simulink model "generic_truck"  (R2025a)
settings: Solver=VariableStepAuto  StartTime=0.0  StopTime=600  FixedStep=0.01  MaxStep=0.001  RelTol=1e-3  EnableMultiTasking=on
libraries: TruckMaker4SL x205, simulink x1
(part 8 of 9)

== matlab function generic_truck/TruckMaker/Tractor_Subsystem /ONE_TRACK_MODEL_TRACTOR_UKF/MATLAB Function1 ==
  data: z input; u input; xhat output; Q input; R input; Ts input; data input; P output; dxdt output; innovation output; K_out output; S_out output; z_pred_out output
function [xhat, P, dxdt, innovation, K_out, S_out, z_pred_out] = UKF_OneTrack_IMU(z, u, Q, R, Ts,data)

persistent x Pk dxdt_old t p_nom Pp

if isempty(x)
    x = [15;0.1;0.1;7.5;7.5];
end
if isempty(Pk)
    Pk = diag([0.1 0.1 0.1 5 5]);
end
if isempty(dxdt_old)
    dxdt_old = zeros(5,1);
end
if isempty(t)
    t = 0;
end
if isempty(p_nom)
    p_nom = [6800; 12994.917];
    Pp = diag([5000, 20000]).^2;
end

T_sim = 0.001;
t = t + T_sim;
t=data;

if t < 30
    xhat = x;
    P = Pk;
    dxdt = dxdt_old;
    innovation = zeros(length(z),1);
    K_out = zeros(length(x), length(z));
    S_out = eye(length(z));
    z_pred_out = zeros(length(z),1);
    return
end

IDX_VX  = 3; 
IDX_WRL = 6; 
IDX_WRR = 7;

g  = 9.82;

p_cog = [3.473;0;0.925];
p_fax = [4.520;0;0.490];
p_rax = [0.950;0;0.490];
p_imu = [3.600;0;1.000];

lf = abs(p_fax(1)-p_cog(1));
lr = abs(p_cog(1)-p_rax(1));
L  = lf + lr;
h  = p_cog(3);

Rfax = p_fax - p_cog; Rfax(3) = -p_cog(3);
Rrax = p_rax - p_cog; Rrax(3) = -p_cog(3);
Rcog = p_imu - p_cog;

delta = u(1);
T_rl  = u(2);
T_rr  = u(3);
Rwheel = 0.505;
Fx_vehicle = (T_rl + T_rr)/Rwheel;

n  = length(x);
np = length(p_nom);
nSPx = 2*n + 1;
nSPp = 2*np;
nSP  = nSPx + nSPp;

W0 = 1 - (n + np)/3;
Wi = (1 - W0)/(2*(n + np));
gamma = sqrt((n + np)/(1 - W0));

%% ===== STATE SIGMA =====
Pk = (Pk + Pk')/2 + 1e-9*eye(n);
Sx = chol(Pk,'lower');

X = zeros(n,nSPx);
X(:,1) = x;
for i=1:n
    X(:,i+1)   = x + gamma*Sx(:,i);
    X(:,i+1+n) = x - gamma*Sx(:,i);
end

%% ===== PARAM SIGMA =====
Pp = (Pp + Pp')/2 + 1e-9*eye(np);
Sp = chol(Pp,'lower');

SPp = zeros(np,nSPp);
for i=1:np
    SPp(:,i)    = p_nom + gamma*Sp(:,i);
    SPp(:,i+np) = p_nom - gamma*Sp(:,i);
end

%% ===== PREDICTION =====
X_prop = zeros(n,nSP);
dxdt_model = zeros(5,1);

for k=1:nSP
    if k <= nSPx
        Xk = X(:,k); 
        pk = p_nom;
    else
        Xk = x; 
        pk = SPp(:,k-nSPx);
    end

    vx=Xk(1); vy=Xk(2); wz=Xk(3); Cf=Xk(4); Cr=Xk(5);
    m=pk(1); Jz=pk(2);

    v_cog=[vx;vy;0]; 
    omega=[0;0;wz];

    Rotf=[cos(delta) -sin(delta) 0;
          sin(delta)  cos(delta)  0; 
           0          0          1];

    vf=Rotf.'*(v_cog+cross(omega,Rfax));
    vr=v_cog+cross(omega,Rrax);

    alpha_f=atan2(vf(2),max(abs(vf(1)),0.1));
    alpha_r=atan2(vr(2),max(abs(vr(1)),0.1));

    ax_est=Fx_vehicle/m+vy*wz;

    Ffz=m*g*lr/L - m*ax_est*h/L;
    Frz=m*g*lf/L + m*ax_est*h/L;

    Fy_f=-Cf*alpha_f*Ffz;
    Fy_r=-Cr*alpha_r*Frz;

    dvx=(Fx_vehicle - Fy_f*sin(delta))/m + vy*wz;
    dvy=(Fy_f*cos(delta)+Fy_r)/m - vx*wz;
    dwz=(lf*Fy_f*cos(delta) - lr*Fy_r)/Jz;

    if k==1
        dxdt_model=[dvx;dvy;dwz;0;0];
    end

    X_prop(:,k)=[vx+Ts*dvx; vy+Ts*dvy; wz+Ts*dwz; Cf; Cr];
end

%% ===== MEAN =====
x_pred=zeros(n,1);
for k=1:nSP
    w=(k==1)*W0 + (k>1)*Wi;
    x_pred=x_pred + w*X_prop(:,k);
end

%% ===== COV =====
P_pred=zeros(n);
for k=1:nSPx
    w=(k==1)*W0 + (k>1)*Wi;
    dx=X_prop(:,k)-x_pred;
    P_pred=P_pred + w*(dx*dx');
end
P_pred=P_pred + Q*Ts;

%% ===== NEW SIGMA POINTS =====
P_pred=(P_pred+P_pred')/2 + 1e-9*eye(n);
Sx=chol(P_pred,'lower');

SPx_new=zeros(n,nSPx);
SPx_new(:,1)=x_pred;

for i=1:n
    SPx_new(:,i+1)  =x_pred+gamma*Sx(:,i);
    SPx_new(:,i+1+n) =x_pred-gamma*Sx(:,i);
end

%% ===== MEASUREMENT =====
Z=zeros(length(z),nSP);

for k=1:nSP
    if k<=nSPx
        Xk=SPx_new(:,k);
        pk=p_nom;
    else
        Xk=x_pred;
        pk=SPp(:,k-nSPx);
    end

    vx=Xk(1); vy=Xk(2); wz=Xk(3);
    Cf=Xk(4); Cr=Xk(5);

    m=pk(1); Jz=pk(2);

    v_cog=[vx;vy;0]; omega=[0;0;wz];
    Rotf=[cos(delta) -sin(delta) 0; sin(delta) cos(delta) 0; 0 0 1];

    vf=Rotf.'*(v_cog+cross(omega,Rfax));
    vr=v_cog+cross(omega,Rrax);

    alpha_f=atan2(vf(2),max(abs(vf(1)),0.1));
    alpha_r=atan2(vr(2),max(abs(vr(1)),0.1));

    ax_est=Fx_vehicle/m+vy*wz;

    Ffz=m*g*lr/L - m*ax_est*h/L;
    Frz=m*g*lf/L + m*ax_est*h/L;

    Fy_f=-Cf*alpha_f*Ffz;
    Fy_r=-Cr*alpha_r*Frz;

    dvx=(Fx_vehicle - Fy_f*sin(delta))/m;
    dvy=(Fy_f*cos(delta)+Fy_r)/m;
    dwz=(lf*Fy_f*cos(delta) - lr*Fy_r)/Jz;

    a_cog=[dvx;dvy;0];
    alpha_vec=[0;0;dwz];

    a_imu=a_cog + cross(omega,cross(omega,Rcog)) + cross(alpha_vec,Rcog);
    v_imu=v_cog + cross(omega,Rcog);

    omega_rl=vx/Rwheel;
    omega_rr=vx/Rwheel;

    Z(:,k)=[a_imu(1:2); v_imu(1:2); wz; omega_rl; omega_rr];
end

%% ===== z mean =====
z_pred=zeros(length(z),1);
for k=1:nSP
    w=(k==1)*W0 + (k>1)*Wi;
    z_pred=z_pred + w*Z(:,k);
end

%% ===== SENSOR SELECTION =====
valid_idx=true(length(z),1);

if ~isnan(z(IDX_VX))
    valid_idx(IDX_WRL)=false;
    valid_idx(IDX_WRR)=false;
else
    valid_idx(IDX_VX)=false;
end

valid_idx=valid_idx & ~isnan(z);

z_used=z(valid_idx);
z_pred_used=z_pred(valid_idx);
Z_used=Z(valid_idx,:);
R_used=R(valid_idx,valid_idx);

%% ===== S =====
S_cov=zeros(length(z_used));
for k=1:nSP
    w=(k==1)*W0 + (k>1)*Wi;
    dz=Z_used(:,k)-z_pred_used;
    S_cov=S_cov + w*(dz*dz');
end

S_cov=S_cov + R_used;
S_cov=(S_cov+S_cov')/2 + 1e-9*eye(size(S_cov));

%% ===== Pxz =====
Pxz=zeros(n,length(z_used));
for k=1:nSPx
    w=(k==1)*W0 + (k>1)*Wi;
    dx=SPx_new(:,k)-x_pred;
    dz=Z_used(:,k)-z_pred_used;
    Pxz=Pxz + w*(dx*dz');
end

%% ===== UPDATE =====
K=Pxz/S_cov;

x=x_pred + K*(z_used - z_pred_used);
Pk=P_pred - K*S_cov*K';
Pk=(Pk+Pk')/2 + 1e-9*eye(n);

%% ===== OUTPUT =====
xhat=x;
P=Pk;
dxdt=dxdt_model;

innovation=zeros(length(z),1);
innovation(valid_idx)=z_used - z_pred_used;

K_out=zeros(n,length(z));
K_out(:,valid_idx)=K;

S_out=zeros(length(z));
S_out(valid_idx,valid_idx)=S_cov;

z_pred_out=z_pred;

end

== matlab function generic_truck/TruckMaker/Tractor_Subsystem /ONE_TRACK_MODEL_TRACTOR_UKF/MATLAB Function2 ==
  data: z input; u input; Q input; R input; Ts input; xhat output; data input; P output; dxdt output; innovation output; K_out output; S_out output; z_pred_out output
function [xhat, P, dxdt, innovation, K_out, S_out, z_pred_out] = UKF_OneTrack_IMU(z, u, Q, R, Ts, data)
z=z(1:5);
persistent x Pk dxdt_old t

%% =========================
%% INIT
%% =========================
if isempty(x)
    % [vx vy wz Cf Cr bax]
    x = [15;0.1;0.1;7.5;7.5;0];
end

if isempty(Pk)
    Pk = diag([0.1 0.1 0.1 5 5 0.5]);
end

if isempty(dxdt_old)
    dxdt_old = zeros(6,1);
end

if isempty(t)
    t = 0;
end

t = data;

if t < 30
    xhat = x;
    P = Pk;
    dxdt = dxdt_old;
    innovation = zeros(length(z),1);
    K_out = zeros(length(x), length(z));
    S_out = eye(length(z));
    z_pred_out = zeros(length(z),1);
    return
end

IDX_VX = 3;
IDX_VY = 4;

%% =========================
%% VEHICLE CONSTANTS
%% =========================
g  = 9.82;

p_cog = [3.473;0;0.925];
p_fax = [4.520;0;0.490];
p_rax = [0.950;0;0.490];
p_imu = [3.600;0;1.000];

lf = abs(p_fax(1)-p_cog(1));
lr = abs(p_cog(1)-p_rax(1));
L  = lf + lr;
h  = p_cog(3);

Rfax = p_fax - p_cog; Rfax(3) = -p_cog(3);
Rrax = p_rax - p_cog; Rrax(3) = -p_cog(3);
Rcog = p_imu - p_cog;

%% =========================
%% INPUTS
%% =========================
delta = u(1);
T_rl  = u(2);
T_rr  = u(3);
Rwheel = 0.505;
Fx_vehicle = (T_rl + T_rr)/Rwheel;

%% =========================
%% UKF PARAMS
%% =========================
n = length(x);
nSPx = 2*n + 1;

W0 = 1 - n/3;
Wi = (1 - W0)/(2*n);
gamma = sqrt(n/(1-W0));

%% =========================
%% SIGMA POINTS (PRIOR)
%% =========================
Pk = (Pk + Pk')/2 + 1e-9*eye(n);
Sx = chol(Pk,'lower');

X_pre = zeros(n,nSPx);
X_pre(:,1) = x;

for i=1:n
    X_pre(:,i+1)   = x + gamma*Sx(:,i);
    X_pre(:,i+1+n) = x - gamma*Sx(:,i);
end

%% =========================
%% PREDICTION
%% =========================
X_pred = zeros(n,nSPx);
dxdt_model = zeros(n,1);

m = 6800; 
Jz = 12994.917;

for k=1:nSPx

    Xk = X_pre(:,k);

    vx = Xk(1); vy = Xk(2); wz = Xk(3);
    Cf = Xk(4); Cr = Xk(5);
    bax = Xk(6);

    v_cog = [vx; vy; 0]; 
    omega = [0; 0; wz];

    Rotf = [cos(delta) -sin(delta) 0;
            sin(delta)  cos(delta) 0;
            0 0 1];

    vf = Rotf.'*(v_cog + cross(omega,Rfax));
    vr = v_cog + cross(omega,Rrax);

    alpha_f = atan2(vf(2), max(abs(vf(1)),0.1));
    alpha_r = atan2(vr(2), max(abs(vr(1)),0.1));

    ax_est = Fx_vehicle/m + vy*wz;

    Ffz = m*g*lr/L - m*ax_est*h/L;
    Frz = m*g*lf/L + m*ax_est*h/L;

    Fy_f = -Cf*alpha_f*Ffz;
    Fy_r = -Cr*alpha_r*Frz;

    dvx = (Fx_vehicle - Fy_f*sin(delta))/m + vy*wz + bax;

    % Testa DÄMPNING här (NYCKELN!)
    dvy = (Fy_f*cos(delta)+Fy_r)/m - vx*wz;

    dwz = (lf*Fy_f*cos(delta) - lr*Fy_r)/Jz;

    if k==1
        dxdt_model = [dvx; dvy; dwz; 0; 0; 0];
    end

    X_pred(:,k) = [
        vx + Ts*dvx
        vy + Ts*dvy
        wz + Ts*dwz
        Cf
        Cr
        bax
    ];
end

%% =========================
%% MEAN
%% =========================
x_pred = zeros(n,1);
for k=1:nSPx
    w = (k==1)*W0 + (k>1)*Wi;
    x_pred = x_pred + w*X_pred(:,k);
end

%% =========================
%% COVARIANCE
%% =========================
P_pred = zeros(n);
for k=1:nSPx
    w = (k==1)*W0 + (k>1)*Wi;
    dx = X_pred(:,k) - x_pred;
    P_pred = P_pred + w*(dx*dx');
end

P_pred = P_pred + Q*Ts;
P_pred = (P_pred + P_pred')/2 + 1e-9*eye(n);

%% =========================
%% SIGMA POINTS (POST)
%% =========================
Sx = chol(P_pred,'lower');

X_post = zeros(n,nSPx);
X_post(:,1) = x_pred;

for i=1:n
    X_post(:,i+1)   = x_pred + gamma*Sx(:,i);
    X_post(:,i+1+n) = x_pred - gamma*Sx(:,i);
end

%% =========================
%% MEASUREMENT MODEL
%% =========================
Z = zeros(length(z), nSPx);

for k=1:nSPx

    Xk = X_post(:,k);

    vx = Xk(1); vy = Xk(2); wz = Xk(3);
    Cf = Xk(4); Cr = Xk(5);
    bax = Xk(6);

    v_cog = [vx; vy; 0]; 
    omega=[0;0;wz];

    Rotf=[cos(delta) -sin(delta) 0;
          sin(delta)  cos(delta) 0;
          0 0 1];

    vf = Rotf.'*(v_cog+cross(omega,Rfax));
    vr = v_cog+cross(omega,Rrax);

    alpha_f = atan2(vf(2), max(abs(vf(1)),0.1));
    alpha_r = atan2(vr(2), max(abs(vr(1)),0.1));

    ax_est = Fx_vehicle/m + vy*wz;

    Ffz = m*g*lr/L - m*ax_est*h/L;
    Frz = m*g*lf/L + m*ax_est*h/L;

    Fy_f = -Cf*alpha_f*Ffz;
    Fy_r = -Cr*alpha_r*Frz;
    
    dvx = (Fx_vehicle - Fy_f*sin(delta))/m;
    dvy = (Fy_f*cos(delta)+Fy_r)/m;
    dwz = (lf*Fy_f*cos(delta) - lr*Fy_r)/Jz;

    a_cog = [dvx; dvy; 0];
    alpha_vec=[0;0;dwz];

    a_imu = a_cog + cross(omega,cross(omega,Rcog)) + cross(alpha_vec,Rcog);
    v_imu = v_cog + cross(omega,Rcog);

    ax_meas = a_imu(1) + bax;

    Z(:,k) = [
        ax_meas
        a_imu(2)
        v_imu(1:2)
        wz
    ];
end

%% =========================
%% MEASUREMENT MEAN
%% =========================
z_pred = zeros(length(z),1);
for k=1:nSPx
    w = (k==1)*W0 + (k>1)*Wi;
    z_pred = z_pred + w*Z(:,k);
end

%% =========================
%% SENSOR SELECTION
%% =========================
valid_idx = true(length(z),1);

if isnan(z(IDX_VX))
    valid_idx(IDX_VX) = false;
    valid_idx(IDX_VY) = false;
end

valid_idx = valid_idx & ~isnan(z);

z_used = z(valid_idx);
z_pred_used = z_pred(valid_idx);
Z_used = Z(valid_idx,:);
R_used = R(valid_idx,valid_idx);

%% =========================
%% S + Pxz
%% =========================
S_cov = zeros(length(z_used));
Pxz = zeros(n,length(z_used));

for k=1:nSPx
    w = (k==1)*W0 + (k>1)*Wi;

    dz = Z_used(:,k)-z_pred_used;
    dx = X_post(:,k)-x_pred;

    S_cov = S_cov + w*(dz*dz');
    Pxz = Pxz + w*(dx*dz');
end

S_cov = S_cov + R_used;
S_cov = (S_cov + S_cov')/2 + 1e-9*eye(size(S_cov));

%% =========================
%% UPDATE
%% =========================
K = Pxz / S_cov;

x = x_pred + K*(z_used - z_pred_used);
Pk = P_pred - K*S_cov*K';
Pk = (Pk + Pk')/2 + 1e-9*eye(n);

%% =========================
%% OUTPUT
%% =========================
xhat = x;
P = Pk;
dxdt = dxdt_model;

innovation = zeros(length(z),1);
innovation(valid_idx) = z_used - z_pred_used;

K_out = zeros(n,length(z));
K_out(:,valid_idx) = K;

S_out = zeros(length(z));
S_out(valid_idx,valid_idx) = S_cov;

z_pred_out = z_pred;

end

== matlab function generic_truck/TruckMaker/Tractor_Subsystem /ONE_TRACK_MODEL_TRACTOR_UKF/UKF_ONE_TRACK1 ==
  data: z input; u input; xhat output; Q input; R input; Ts input; P output; dxdt output; innovation output; K_out output; S_out output; z_pred_out output; data input
function [xhat, P, dxdt, innovation, K_out, S_out, z_pred_out] = UKF_OneTrack_IMU(z, u, Q, R, Ts,data)

persistent x Pk dxdt_old t p_nom Pp

if isempty(x)
    x = [15;0.1;0.1;7.5;7.5];
end
if isempty(Pk)
    Pk = diag([0.1 0.1 0.1 5 5]);
end
if isempty(dxdt_old)
    dxdt_old = zeros(5,1);
end
if isempty(t)
    t = 0;
end
if isempty(p_nom)
    p_nom = [6800; 12994.917];
    Pp = diag([5000, 20000]).^2;
end

T_sim = 0.001;
t = t + T_sim;
t=data;

if t < 49.9
    xhat = x;
    P = Pk;
    dxdt = dxdt_old;
    innovation = zeros(length(z),1);
    K_out = zeros(length(x), length(z));
    S_out = eye(length(z));
    z_pred_out = zeros(length(z),1);
    return
end

IDX_VX  = 3; 
IDX_WRL = 6; 
IDX_WRR = 7;

g  = 9.82;

p_cog = [3.473;0;0.925];
p_fax = [4.520;0;0.490];
p_rax = [0.950;0;0.490];
p_imu = [3.600;0;1.000];

lf = abs(p_fax(1)-p_cog(1));
lr = abs(p_cog(1)-p_rax(1));
L  = lf + lr;
h  = p_cog(3);

Rfax = p_fax - p_cog; Rfax(3) = -p_cog(3);
Rrax = p_rax - p_cog; Rrax(3) = -p_cog(3);
Rcog = p_imu - p_cog;

delta = u(1);
T_rl  = u(2);
T_rr  = u(3);
F_brake= abs(u(4)) + abs(u(5));
Rwheel = 0.505;
Fx_vehicle = (T_rl + T_rr)/Rwheel - F_brake;

n  = length(x);
np = length(p_nom);
nSPx = 2*n + 1;
nSPp = 2*np;
nSP  = nSPx + nSPp;

W0 = 1 - (n + np)/3;
Wi = (1 - W0)/(2*(n + np));
gamma = sqrt((n + np)/(1 - W0));

%% ===== STATE SIGMA =====
Pk = (Pk + Pk')/2 + 1e-9*eye(n);
Sx = chol(Pk,'lower');

X = zeros(n,nSPx);
X(:,1) = x;
for i=1:n
    X(:,i+1)   = x + gamma*Sx(:,i);
    X(:,i+1+n) = x - gamma*Sx(:,i);
end

%% ===== PARAM SIGMA =====
Pp = (Pp + Pp')/2 + 1e-9*eye(np);
Sp = chol(Pp,'lower');

SPp = zeros(np,nSPp);
for i=1:np
    SPp(:,i)    = p_nom + gamma*Sp(:,i);
    SPp(:,i+np) = p_nom - gamma*Sp(:,i);
end

%% ===== PREDICTION =====
X_prop = zeros(n,nSP);
dxdt_model = zeros(5,1);

for k=1:nSP
    if k <= nSPx
        Xk = X(:,k); 
        pk = p_nom;
    else
        Xk = x; 
        pk = SPp(:,k-nSPx);
    end

    vx=Xk(1); vy=Xk(2); wz=Xk(3); Cf=Xk(4); Cr=Xk(5);
    m=pk(1); Jz=pk(2);

    v_cog=[vx;vy;0]; omega=[0;0;wz];
    Rotf=[cos(delta) -sin(delta) 0; sin(delta) cos(delta) 0; 0 0 1];

    vf=Rotf.'*(v_cog+cross(omega,Rfax));
    vr=v_cog+cross(omega,Rrax);

    alpha_f=atan2(vf(2),max(abs(vf(1)),0.1));
    alpha_r=atan2(vr(2),max(abs(vr(1)),0.1));

    ax_est=Fx_vehicle/m+vy*wz;

    Ffz=m*g*lr/L - m*ax_est*h/L;
    Frz=m*g*lf/L + m*ax_est*h/L;

    Fy_f=-Cf*alpha_f*Ffz;
    Fy_r=-Cr*alpha_r*Frz;

    dvx=(Fx_vehicle - Fy_f*sin(delta))/m + vy*wz;
    dvy=(Fy_f*cos(delta)+Fy_r)/m - vx*wz;
    dwz=(lf*Fy_f*cos(delta) - lr*Fy_r)/Jz;

    if k==1
        dxdt_model=[dvx;dvy;dwz;0;0];
    end

    X_prop(:,k)=[vx+Ts*dvx; vy+Ts*dvy; wz+Ts*dwz; Cf; Cr];
end

%% ===== MEAN =====
x_pred=zeros(n,1);
for k=1:nSP
    w=(k==1)*W0 + (k>1)*Wi;
    x_pred=x_pred + w*X_prop(:,k);
end

%% ===== COV =====
P_pred=zeros(n);
for k=1:nSPx
    w=(k==1)*W0 + (k>1)*Wi;
    dx=X_prop(:,k)-x_pred;
    P_pred=P_pred + w*(dx*dx');
end
P_pred=P_pred + Q*Ts;

%% ===== NEW SIGMA POINTS =====
P_pred=(P_pred+P_pred')/2 + 1e-9*eye(n);
Sx=chol(P_pred,'lower');

SPx_new=zeros(n,nSPx);
SPx_new(:,1)=x_pred;

for i=1:n
    SPx_new(:,i+1)=x_pred+gamma*Sx(:,i);
    SPx_new(:,i+1+n)=x_pred-gamma*Sx(:,i);
end

%% ===== MEASUREMENT =====
Z=zeros(length(z),nSP);

for k=1:nSP
    if k<=nSPx
        Xk=SPx_new(:,k);
        pk=p_nom;
    else
        Xk=x_pred;
        pk=SPp(:,k-nSPx);
    end

    vx=Xk(1); vy=Xk(2); wz=Xk(3);
    Cf=Xk(4); Cr=Xk(5);

    m=pk(1); Jz=pk(2);

    v_cog=[vx;vy;0]; omega=[0;0;wz];
    Rotf=[cos(delta) -sin(delta) 0; sin(delta) cos(delta) 0; 0 0 1];

    vf=Rotf.'*(v_cog+cross(omega,Rfax));
    vr=v_cog+cross(omega,Rrax);

    alpha_f=atan2(vf(2),max(abs(vf(1)),0.1));
    alpha_r=atan2(vr(2),max(abs(vr(1)),0.1));

    ax_est=Fx_vehicle/m+vy*wz;

    Ffz=m*g*lr/L - m*ax_est*h/L;
    Frz=m*g*lf/L + m*ax_est*h/L;

    Fy_f=-Cf*alpha_f*Ffz;
    Fy_r=-Cr*alpha_r*Frz;

    dvx=(Fx_vehicle - Fy_f*sin(delta))/m;
    dvy=(Fy_f*cos(delta)+Fy_r)/m;
    dwz=(lf*Fy_f*cos(delta) - lr*Fy_r)/Jz;

    a_cog=[dvx;dvy;0];
    alpha_vec=[0;0;dwz];

    a_imu=a_cog + cross(omega,cross(omega,Rcog)) + cross(alpha_vec,Rcog);
    v_imu=v_cog + cross(omega,Rcog);

    omega_rl=vx/Rwheel;
    omega_rr=vx/Rwheel;

    Z(:,k)=[a_imu(1:2); v_imu(1:2); wz; omega_rl; omega_rr];
end

%% ===== z mean =====
z_pred=zeros(length(z),1);
for k=1:nSP
    w=(k==1)*W0 + (k>1)*Wi;
    z_pred=z_pred + w*Z(:,k);
end

%% ===== SENSOR SELECTION =====
valid_idx=true(length(z),1);

if ~isnan(z(IDX_VX))
    valid_idx(IDX_WRL)=false;
    valid_idx(IDX_WRR)=false;
else
    valid_idx(IDX_VX)=false;
end

valid_idx=valid_idx & ~isnan(z);

z_used=z(valid_idx);
z_pred_used=z_pred(valid_idx);
Z_used=Z(valid_idx,:);
R_used=R(valid_idx,valid_idx);

%% ===== S =====
S_cov=zeros(length(z_used));
for k=1:nSP
    w=(k==1)*W0 + (k>1)*Wi;
    dz=Z_used(:,k)-z_pred_used;
    S_cov=S_cov + w*(dz*dz');
end

S_cov=S_cov + R_used;
S_cov=(S_cov+S_cov')/2 + 1e-9*eye(size(S_cov));

%% ===== Pxz =====
Pxz=zeros(n,length(z_used));
for k=1:nSPx
    w=(k==1)*W0 + (k>1)*Wi;
    dx=SPx_new(:,k)-x_pred;
    dz=Z_used(:,k)-z_pred_used;
    Pxz=Pxz + w*(dx*dz');
end

%% ===== UPDATE =====
K=Pxz/S_cov;

x=x_pred + K*(z_used - z_pred_used);
Pk=P_pred - K*S_cov*K';
Pk=(Pk+Pk')/2 + 1e-9*eye(n);

%% ===== OUTPUT =====
xhat=x;
P=Pk;
dxdt=dxdt_model;

innovation=zeros(length(z),1);
innovation(valid_idx)=z_used - z_pred_used;

K_out=zeros(n,length(z));
K_out(:,valid_idx)=K;

S_out=zeros(length(z));
S_out(valid_idx,valid_idx)=S_cov;

z_pred_out=z_pred;

end

== matlab function generic_truck/TruckMaker/Tractor_Subsystem /ONE_TRACK_MODEL_TRACTOR_UKF/Working Model with 5 measurements  ==
  data: z input; u input; xhat output; Q input; R input; Ts input; P output; dxdt output; innovation output; K_out output; S_out output; z_pred_out output
function [xhat, P, dxdt, innovation, K_out, S_out, z_pred_out] = UKF_OneTrack_IMU(z, u, Q, R, Ts)

% z = [ax; ay; vx; vy; wz]

%% =========================
%% PERSISTENT VARIABLES
%% =========================
persistent x Pk dxdt_old t

if isempty(x)
    x = [15;0.1;0.1;7.5;7.5];   % [vx vy wz Cf Cr]
end
if isempty(Pk)
    Pk = diag([0.1 0.1 0.1 2 2]);
end
if isempty(dxdt_old)
    dxdt_old = zeros(5,1);
end
if isempty(t)
    t = 0;
end

%% =========================
%% TIME UPDATE
%% =========================
t = t + 0.001;

start_time = 30;
if t < start_time
    xhat = x;
    P = Pk;
    dxdt = dxdt_old;

    innovation = zeros(length(z),1);
    K_out = zeros(length(x), length(z));
    S_out = eye(length(z));
    z_pred_out = zeros(length(z),1);
    return
end

%% =========================
%% VEHICLE PARAMETERS
%% =========================
m  = 6800;
g  = 9.82;
Jz = 12994.917;

p_cog = [3.473;0;0.925];
p_fax = [4.520;0;0.490];
p_rax = [0.950;0;0.490];
p_imu = [3.600;0;1.000];

lf = abs(p_fax(1)-p_cog(1));
lr = abs(p_cog(1)-p_rax(1));
L  = lf + lr;
h  = p_cog(3);

Rfax = p_fax - p_cog; Rfax(3) = -p_cog(3);
Rrax = p_rax - p_cog; Rrax(3) = -p_cog(3);
Rcog = p_imu - p_cog;

%% =========================
%% INPUTS
%% =========================
delta = u(1);
T_rl  = u(2);
T_rr  = u(3);
Rwheel = 0.505;

Fx_vehicle = (T_rl + T_rr)/(Rwheel);

%% =========================
%% UKF PARAMETERS
%% =========================
n = length(x);
W0 = 1 - n/3;
Wi = (1 - W0)/(2*n);
gamma = sqrt(n/(1-W0));

Pk = (Pk+Pk')/2 + 1e-9*eye(n);
S = chol(Pk,'lower');

%% =========================
%% SIGMA POINTS
%% =========================
X = zeros(n,2*n+1);
X(:,1) = x;

for i=1:n
    X(:,i+1)   = x + gamma*S(:,i);
    X(:,i+1+n) = x - gamma*S(:,i);
end

%% =========================
%% PREDICTION
%% =========================
X_pred = zeros(n,2*n+1);
dxdt_model = zeros(5,1);

for k=1:2*n+1

    vx = X(1,k);
    vy = X(2,k);
    wz = X(3,k);
    Cf = X(4,k);
    Cr = X(5,k);

    v_cog = [vx;vy;0];
    omega = [0;0;wz];

    Rotf = [cos(delta) -sin(delta) 0;
            sin(delta)  cos(delta) 0;
            0 0 1];

    vf = Rotf.'*(v_cog + cross(omega,Rfax));
    vr = v_cog + cross(omega,Rrax);

    alpha_f = atan2(vf(2), max(abs(vf(1)),0.1));
    alpha_r = atan2(vr(2), max(abs(vr(1)),0.1));

    ax_est = Fx_vehicle/m + vy*wz;

    Ffz = m*g*lr/L - m*ax_est*h/L;
    Frz = m*g*lf/L + m*ax_est*h/L;

    Fy_f = -Cf * alpha_f * Ffz;
    Fy_r = -Cr * alpha_r * Frz;

    dvx = (Fx_vehicle - Fy_f*sin(delta))/m + vy*wz;
    dvy = (Fy_f*cos(delta) + Fy_r)/m - vx*wz;
    dwz = (lf*Fy_f*cos(delta) - lr*Fy_r)/Jz;

    if k==1
        dxdt_model = [dvx; dvy; dwz; 0; 0];
    end

    X_pred(:,k) = [
        vx + Ts*dvx
        vy + Ts*dvy
        wz + Ts*dwz
        Cf
        Cr
    ];
end

%% =========================
%% MEAN + COV
%% =========================
x_pred = W0*X_pred(:,1);
for k=2:2*n+1
    x_pred = x_pred + Wi*X_pred(:,k);
end

P_pred = zeros(n);
for k=1:2*n+1
    w = (k==1)*W0 + (k>1)*Wi;
    dx = X_pred(:,k)-x_pred;
    P_pred = P_pred + w*(dx*dx');
end
P_pred = P_pred + Q*Ts;

%% =========================
%% MEASUREMENT MODEL
%% =========================
Z = zeros(length(z),2*n+1);

for k=1:2*n+1

    vx = X_pred(1,k);
    vy = X_pred(2,k);
    wz = X_pred(3,k);
    Cf = X_pred(4,k);
    Cr = X_pred(5,k);

    v_cog = [vx;vy;0];
    omega = [0;0;wz];

    Rotf = [cos(delta) -sin(delta) 0;
            sin(delta)  cos(delta) 0;
            0 0 1];

    vf = Rotf.'*(v_cog + cross(omega,Rfax));
    vr = v_cog + cross(omega,Rrax);

    alpha_f = atan2(vf(2), max(abs(vf(1)),0.1));
    alpha_r = atan2(vr(2), max(abs(vr(1)),0.1));

    ax_est = Fx_vehicle/m + vy*wz;

    Ffz = m*g*lr/L - m*ax_est*h/L;
    Frz = m*g*lf/L + m*ax_est*h/L;

    Fy_f = -Cf * alpha_f * Ffz;
    Fy_r = -Cr * alpha_r * Frz;

    dvx = (Fx_vehicle - Fy_f*sin(delta))/m;
    dvy = (Fy_f*cos(delta) + Fy_r)/m;
    dwz = (lf*Fy_f*cos(delta) - lr*Fy_r)/Jz;

    a_cog = [dvx; dvy; 0];
    alpha_vec = [0;0;dwz];

    a_imu = a_cog + cross(omega,cross(omega,Rcog)) + cross(alpha_vec,Rcog);
    v_imu = v_cog + cross(omega,Rcog);

    Z(:,k) = [a_imu(1:2); v_imu(1:2); wz];
end

%% =========================
%% HANDLE NaN MEASUREMENTS
%% =========================
valid_idx = ~isnan(z);

z_used      = z(valid_idx);
z_pred      = W0*Z(:,1);
for k=2:2*n+1
    z_pred = z_pred + Wi*Z(:,k);
end

z_pred_used = z_pred(valid_idx);
Z_used      = Z(valid_idx,:);
R_used      = R(valid_idx, valid_idx);

%% =========================
%% S
%% =========================
S_cov = zeros(length(z_used));
for k=1:2*n+1
    w = (k==1)*W0 + (k>1)*Wi;
    dz = Z_used(:,k)-z_pred_used;
    S_cov = S_cov + w*(dz*dz');
end
S_cov = S_cov + R_used;

%% =========================
%% Pxz
%% =========================
Pxz = zeros(n,length(z_used));
for k=1:2*n+1
    w = (k==1)*W0 + (k>1)*Wi;
    dx = X_pred(:,k)-x_pred;
    dz = Z_used(:,k)-z_pred_used;
    Pxz = Pxz + w*(dx*dz');
end

%% =========================
%% UPDATE
%% =========================
K = Pxz / S_cov;

x = x_pred + K*(z_used - z_pred_used);
Pk = P_pred - K*S_cov*K';
Pk = (Pk+Pk')/2 + 1e-9*eye(n);

%% =========================
%% OUTPUTS
%% =========================
dxdt_old = dxdt_model;

xhat = x;
P = Pk;
dxdt = dxdt_old;

innovation = zeros(length(z),1);
innovation(valid_idx) = z_used - z_pred_used;

K_out = zeros(n,length(z));
K_out(:,valid_idx) = K;

S_out = zeros(length(z));
S_out(valid_idx,valid_idx) = S_cov;

z_pred_out = z_pred;

end

== matlab function generic_truck/TruckMaker/Tractor_Subsystem /ONE_TRACK_MODEL_TRACTOR_UKF/Working Model with 7 measurements ==
  data: z input; u input; xhat output; Q input; R input; Ts input; P output; dxdt output; innovation output; K_out output; S_out output; z_pred_out output; data input
function [xhat, P, dxdt, innovation, K_out, S_out, z_pred_out] = UKF_OneTrack_IMU(z, u, Q, R, Ts,data)

persistent x Pk dxdt_old t p_nom Pp

if isempty(x)
    x = [15;0.1;0.1;7.5;7.5];
end
if isempty(Pk)
    Pk = diag([0.1 0.1 0.1 5 5]);
end
if isempty(dxdt_old)
    dxdt_old = zeros(5,1);
end
if isempty(t)
    t = 0;
end
if isempty(p_nom)
    p_nom = [6800; 12994.917];
    Pp = diag([5000, 20000]).^2;
end

T_sim = 0.001;
t = t + T_sim;
t=data;

if t < 30
    xhat = x;
    P = Pk;
    dxdt = dxdt_old;
    innovation = zeros(length(z),1);
    K_out = zeros(length(x), length(z));
    S_out = eye(length(z));
    z_pred_out = zeros(length(z),1);
    return
end

IDX_VX  = 3; 
IDX_WRL = 6; 
IDX_WRR = 7;

g  = 9.82;

p_cog = [3.473;0;0.925];
p_fax = [4.520;0;0.490];
p_rax = [0.950;0;0.490];
p_imu = [3.600;0;1.000];

lf = abs(p_fax(1)-p_cog(1));
lr = abs(p_cog(1)-p_rax(1));
L  = lf + lr;
h  = p_cog(3);

Rfax = p_fax - p_cog; Rfax(3) = -p_cog(3);
Rrax = p_rax - p_cog; Rrax(3) = -p_cog(3);
Rcog = p_imu - p_cog;

delta = u(1);
T_rl  = u(2);
T_rr  = u(3);
Rwheel = 0.505;
Fx_vehicle = (T_rl + T_rr)/Rwheel;

n  = length(x);
np = length(p_nom);
nSPx = 2*n + 1;
nSPp = 2*np;
nSP  = nSPx + nSPp;

W0 = 1 - (n + np)/3;
Wi = (1 - W0)/(2*(n + np));
gamma = sqrt((n + np)/(1 - W0));

%% ===== STATE SIGMA =====
Pk = (Pk + Pk')/2 + 1e-9*eye(n);
Sx = chol(Pk,'lower');

X = zeros(n,nSPx);
X(:,1) = x;
for i=1:n
    X(:,i+1)   = x + gamma*Sx(:,i);
    X(:,i+1+n) = x - gamma*Sx(:,i);
end

%% ===== PARAM SIGMA =====
Pp = (Pp + Pp')/2 + 1e-9*eye(np);
Sp = chol(Pp,'lower');

SPp = zeros(np,nSPp);
for i=1:np
    SPp(:,i)    = p_nom + gamma*Sp(:,i);
    SPp(:,i+np) = p_nom - gamma*Sp(:,i);
end

%% ===== PREDICTION =====
X_prop = zeros(n,nSP);
dxdt_model = zeros(5,1);

for k=1:nSP
    if k <= nSPx
        Xk = X(:,k); 
        pk = p_nom;
    else
        Xk = x; 
        pk = SPp(:,k-nSPx);
    end

    vx=Xk(1); vy=Xk(2); wz=Xk(3); Cf=Xk(4); Cr=Xk(5);
    m=pk(1); Jz=pk(2);

    v_cog=[vx;vy;0]; omega=[0;0;wz];
    Rotf=[cos(delta) -sin(delta) 0; sin(delta) cos(delta) 0; 0 0 1];

    vf=Rotf.'*(v_cog+cross(omega,Rfax));
    vr=v_cog+cross(omega,Rrax);

    alpha_f=atan2(vf(2),max(abs(vf(1)),0.1));
    alpha_r=atan2(vr(2),max(abs(vr(1)),0.1));

    ax_est=Fx_vehicle/m+vy*wz;

    Ffz=m*g*lr/L - m*ax_est*h/L;
    Frz=m*g*lf/L + m*ax_est*h/L;

    Fy_f=-Cf*alpha_f*Ffz;
    Fy_r=-Cr*alpha_r*Frz;

    dvx=(Fx_vehicle - Fy_f*sin(delta))/m + vy*wz;
    dvy=(Fy_f*cos(delta)+Fy_r)/m - vx*wz;
    dwz=(lf*Fy_f*cos(delta) - lr*Fy_r)/Jz;

    if k==1
        dxdt_model=[dvx;dvy;dwz;0;0];
    end

    X_prop(:,k)=[vx+Ts*dvx; vy+Ts*dvy; wz+Ts*dwz; Cf; Cr];
end

%% ===== MEAN =====
x_pred=zeros(n,1);
for k=1:nSP
    w=(k==1)*W0 + (k>1)*Wi;
    x_pred=x_pred + w*X_prop(:,k);
end

%% ===== COV =====
P_pred=zeros(n);
for k=1:nSPx
    w=(k==1)*W0 + (k>1)*Wi;
    dx=X_prop(:,k)-x_pred;
    P_pred=P_pred + w*(dx*dx');
end
P_pred=P_pred + Q*Ts;

%% ===== NEW SIGMA POINTS =====
P_pred=(P_pred+P_pred')/2 + 1e-9*eye(n);
Sx=chol(P_pred,'lower');

SPx_new=zeros(n,nSPx);
SPx_new(:,1)=x_pred;

for i=1:n
    SPx_new(:,i+1)=x_pred+gamma*Sx(:,i);
    SPx_new(:,i+1+n)=x_pred-gamma*Sx(:,i);
end

%% ===== MEASUREMENT =====
Z=zeros(length(z),nSP);

for k=1:nSP
    if k<=nSPx
        Xk=SPx_new(:,k);
        pk=p_nom;
    else
        Xk=x_pred;
        pk=SPp(:,k-nSPx);
    end

    vx=Xk(1); vy=Xk(2); wz=Xk(3);
    Cf=Xk(4); Cr=Xk(5);

    m=pk(1); Jz=pk(2);

    v_cog=[vx;vy;0]; omega=[0;0;wz];
    Rotf=[cos(delta) -sin(delta) 0; sin(delta) cos(delta) 0; 0 0 1];

    vf=Rotf.'*(v_cog+cross(omega,Rfax));
    vr=v_cog+cross(omega,Rrax);

    alpha_f=atan2(vf(2),max(abs(vf(1)),0.1));
    alpha_r=atan2(vr(2),max(abs(vr(1)),0.1));

    ax_est=Fx_vehicle/m+vy*wz;

    Ffz=m*g*lr/L - m*ax_est*h/L;
    Frz=m*g*lf/L + m*ax_est*h/L;

    Fy_f=-Cf*alpha_f*Ffz;
    Fy_r=-Cr*alpha_r*Frz;

    dvx=(Fx_vehicle - Fy_f*sin(delta))/m;
    dvy=(Fy_f*cos(delta)+Fy_r)/m;
    dwz=(lf*Fy_f*cos(delta) - lr*Fy_r)/Jz;

    a_cog=[dvx;dvy;0];
    alpha_vec=[0;0;dwz];

    a_imu=a_cog + cross(omega,cross(omega,Rcog)) + cross(alpha_vec,Rcog);
    v_imu=v_cog + cross(omega,Rcog);

    omega_rl=vx/Rwheel;
    omega_rr=vx/Rwheel;

    Z(:,k)=[a_imu(1:2); v_imu(1:2); wz; omega_rl; omega_rr];
end

%% ===== z mean =====
z_pred=zeros(length(z),1);
for k=1:nSP
    w=(k==1)*W0 + (k>1)*Wi;
    z_pred=z_pred + w*Z(:,k);
end

%% ===== SENSOR SELECTION =====
valid_idx=true(length(z),1);

if ~isnan(z(IDX_VX))
    valid_idx(IDX_WRL)=false;
    valid_idx(IDX_WRR)=false;
else
    valid_idx(IDX_VX)=false;
end

valid_idx=valid_idx & ~isnan(z);

z_used=z(valid_idx);
z_pred_used=z_pred(valid_idx);
Z_used=Z(valid_idx,:);
R_used=R(valid_idx,valid_idx);

%% ===== S =====
S_cov=zeros(length(z_used));
for k=1:nSP
    w=(k==1)*W0 + (k>1)*Wi;
    dz=Z_used(:,k)-z_pred_used;
    S_cov=S_cov + w*(dz*dz');
end

S_cov=S_cov + R_used;
S_cov=(S_cov+S_cov')/2 + 1e-9*eye(size(S_cov));

%% ===== Pxz =====
Pxz=zeros(n,length(z_used));
for k=1:nSPx
    w=(k==1)*W0 + (k>1)*Wi;
    dx=SPx_new(:,k)-x_pred;
    dz=Z_used(:,k)-z_pred_used;
    Pxz=Pxz + w*(dx*dz');
end

%% ===== UPDATE =====
K=Pxz/S_cov;

x=x_pred + K*(z_used - z_pred_used);
Pk=P_pred - K*S_cov*K';
Pk=(Pk+Pk')/2 + 1e-9*eye(n);

%% ===== OUTPUT =====
xhat=x;
P=Pk;
dxdt=dxdt_model;

innovation=zeros(length(z),1);
innovation(valid_idx)=z_used - z_pred_used;

K_out=zeros(n,length(z));
K_out(:,valid_idx)=K;

S_out=zeros(length(z));
S_out(valid_idx,valid_idx)=S_cov;

z_pred_out=z_pred;

end

== matlab function generic_truck/TruckMaker/Tractor_Subsystem /Subsystem/Ackerman Angle/MATLAB Function ==
  data: delta_l input; delta output; delta_r input
function delta = ackerman_angle(delta_l, delta_r)

delta = acot((cot(delta_l) + cot(delta_r))/2);

end

== matlab function generic_truck/TruckMaker/Tractor_Subsystem /Subsystem_Noisey Measurements/MATLAB Function ==
  data: gyro_true input; gyro_meas output
function gyro_meas = imu_gyro_noise(gyro_true)

Fs = 1000;   % sample rate

[meas, ~] = GyroNoise(gyro_true', Fs);

gyro_meas = meas';

end

== matlab function generic_truck/TruckMaker/Tractor_Subsystem /Subsystem_Noisey Measurements/MATLAB Function1 ==
  data: acc_true input; acc_meas output
function acc_meas = AccelNoiseBlock(acc_true)

Fs = 1000;

truth = acc_true;      % 1×3

[meas,~] = AccelNoise(truth,Fs);

acc_meas = meas;       % 3×1

end

== matlab function generic_truck/TruckMaker/Tractor_Subsystem /Subsystem_Noisey Measurements/MATLAB Function2 ==
  data: truth input; vel_meas output
function vel_meas = imu_vel_noise(truth)
    

sigma = 0.05; % m/s^2 (tune later)

vel_meas = truth + sigma * randn(size(truth));


end

== matlab function generic_truck/TruckMaker/Tractor_Subsystem /Subsystem_Noisey Measurements _NAN/MATLAB Function3 ==
  data: truth input; vel_meas output
function vel_meas = imu_vel_noise(truth)
    

sigma = 0.05; % m/s^2 (tune later)

vel_meas = truth + sigma * randn(size(truth));


end

== matlab function generic_truck/TruckMaker/Tractor_Subsystem /Subsystem_Noisey Measurements _NAN/MATLAB Function ==
  data: gyro_true input; gyro_meas output
function gyro_meas = imu_gyro_noise(gyro_true)

Fs = 1000;   % sample rate

[meas, ~] = GyroNoise(gyro_true', Fs);

gyro_meas = meas';

end

== matlab function generic_truck/TruckMaker/Tractor_Subsystem /Subsystem_Noisey Measurements _NAN/MATLAB Function1 ==
  data: acc_true input; acc_meas output
function acc_meas = AccelNoiseBlock(acc_true)

Fs = 1000;

truth = acc_true;      % 1×3

[meas,~] = AccelNoise(truth,Fs);

acc_meas = meas;       % 3×1

end

== matlab function generic_truck/TruckMaker/Tractor_Subsystem /Subsystem_Noisey Measurements _NAN/MATLAB Function2 ==
  data: truth input; vel_meas output
function vel_meas = imu_vel_noise(truth)
    

sigma = 0.05; % m/s^2 (tune later)

vel_meas = truth + sigma * randn(size(truth));


end

== matlab function generic_truck/TruckMaker/Tractor_Subsystem /Subsystem_Noisey Measurements/MATLAB Function3 ==
  data: truth input; vel_meas output
function vel_meas = imu_vel_noise(truth)
    

sigma = 0.05; % m/s^2 (tune later)

vel_meas = truth + sigma * randn(size(truth));


end

== matlab function generic_truck/TruckMaker/Two_TRack_Model/MATLAB Function1 ==
  data: z input; u input; xhat output; Q input; R input; Ts input; P output
function [xhat, P] = CKF_Bicycle_IPG(z, u, Q, R, Ts)
% Cubature Kalman Filter for One-Track vehicle model
% States: [vx vy r Cf Cr]'
% Measurements: [ay r vx]'

% -------------------------------------------------
% Persistent states (SIMULINK SAFE)
% -------------------------------------------------
persistent x Pk

if isempty(x)
    x  = [15; 0; 0.05; 6e4; 6e4];
    Pk = diag([1 1 0.05 2e4 2e4].^2);
end

n = length(x);   % state dimension
m = length(z);   % measurement dimension

% -------------------------------------------------
% Cubature points
% -------------------------------------------------
Xi = sqrt(n) * [eye(n) -eye(n)];
W  = ones(1,2*n) / (2*n);

% -------------------------------------------------
% PREDICTION STEP
% -------------------------------------------------
X_pred = zeros(n,2*n);
S = chol(Pk,'lower');

for i = 1:2*n
    X_sigma = x + S*Xi(:,i);
    X_pred(:,i) = VehicleDynamics(X_sigma, u, Ts);
end

x_pred = X_pred * W';

P_pred = Q;
for i = 1:2*n
    dx = X_pred(:,i) - x_pred;
    P_pred = P_pred + W(i) * (dx*dx');
end

% -------------------------------------------------
% MEASUREMENT PREDICTION
% -------------------------------------------------
Z_sigma = zeros(m,2*n);
for i = 1:2*n
    Z_sigma(:,i) = MeasurementModel(X_pred(:,i), u);
end

z_pred = Z_sigma * W';

Pzz = R;
Pxz = zeros(n,m);
for i = 1:2*n
    dz = Z_sigma(:,i) - z_pred;
    dx = X_pred(:,i) - x_pred;
    Pzz = Pzz + W(i)*(dz*dz');
    Pxz = Pxz + W(i)*(dx*dz');
end

% -------------------------------------------------
% UPDATE STEP
% -------------------------------------------------
K = Pxz / Pzz;

x  = x_pred + K*(z - z_pred);
Pk = P_pred - K*Pzz*K';

xhat = x;
P    = Pk;

end
function x_next = VehicleDynamics(x, u, Ts)

% States
vx = x(1); vy = x(2); r = x(3);
Cf = x(4); Cr = x(5);

% Inputs
delta = u(1);    % steering angle [rad]
Fx    = u(2);    % longitudinal force [N]

% Vehicle parameters
m  = 7000;
Jz = 14232;
lf = 1.12;
lr = 2.45;

vx_eff = max(abs(vx), 3);

% Slip angles
alpha_f = (vy + lf*r)/vx_eff - delta;
alpha_r = (vy - lr*r)/vx_eff;

% Tire forces
Fyf = -Cf * alpha_f;
Fyr = -Cr * alpha_r;

% Dynamics
dvx = (Fx - Fyf*sin(delta) + vy*r)/m;
dvy = (Fyf*cos(delta) + Fyr - vx*r)/m;
dr  = (lf*Fyf*cos(delta) - lr*Fyr)/Jz;

% Parameters as random walk
dCf = 0;
dCr = 0;

% Euler integration
x_next = x + Ts*[dvx; dvy; dr; dCf; dCr];

end
function z = MeasurementModel(x, u)

vx = x(1); vy = x(2); r = x(3);
Cf = x(4); Cr = x(5);
delta = u(1);

% Vehicle parameters
m  = 7000;
lf = 1.12;
lr = 2.45;

vx_eff = max(abs(vx),3);

% Slip angles
alpha_f = (vy + lf*r)/vx_eff - delta;
alpha_r = (vy - lr*r)/vx_eff;

% Tire forces
Fyf = -Cf * alpha_f;
Fyr = -Cr * alpha_r;

% Lateral acceleration (IMU)
dvy = (Fyf*cos(delta) + Fyr - vx*r)/m;
ay  = dvy + vx*r;

% Measurement vector
z = [
    ay
    r
    vx
];

end

== matlab function generic_truck/TruckMaker/Two_TRack_Model/MATLAB Function ==
  data: z input; u input; xhat output; Q input; R input; Ts input; P output
function [xhat, P] = EKF_Bicycle_Full_NoBias(z, u, Q, R, Ts)
% EKF for One-Track / Bicycle Model (No IMU Bias)
% States: x = [vx; vy; r; Cf; Cr]
% Measurements: z = [ax; ay; vx; vy; r; wL; wR]

persistent x Pk
if isempty(x)
    % Initial state guess
    x = [15; 0; 0.05; 6e4; 6e4]; % vx, vy, r, Cf, Cr
    Pk = diag([1 1 0.05 2e4 2e4].^2);
end

%% Vehicle parameters
m  = 7000;       % mass
Jz = 14232;      % yaw inertia
lf = 1.12;       % front CG distance
lr = 2.45;       % rear CG distance
Rw = 0.49;       % wheel radius
track = 2.49;    % track width

%% Inputs
delta = u(1); % steering angle
Fx = u(2);    % longitudinal force

%% States
vx = x(1); vy = x(2); r = x(3);
Cf = x(4); Cr = x(5);

%% Protect low velocity
vx_eff = max(abs(vx), 3);

%% ---------------- Prediction ----------------
% Slip angles
alpha_f = (vy + lf*r)/vx_eff - delta;
alpha_r = (vy - lr*r)/vx_eff;

% Tire lateral forces
Fyf = -Cf*alpha_f; % Cyf= FyF/slip
Fyr = -Cr*alpha_r;

% Vehicle dynamics
dvx = (Fx - Fyf*sin(delta) + vy*r)/m;
dvy = (Fyf*cos(delta) + Fyr - vx*r)/m;
dr  = (lf*Fyf*cos(delta) - lr*Fyr)/Jz;

% State propagation
xdot = [dvx; dvy; dr; 0; 0];
x_pred = x + Ts*xdot;

%% ---------------- Jacobian F ----------------
F = eye(5);

% Partial derivatives for F
% alpha derivatives
dalf_dvx = -(vy + lf*r)/vx_eff^2;
dalf_dvy = 1/vx_eff;
dalf_dr  = lf/vx_eff;

dalr_dvx = -(vy - lr*r)/vx_eff^2;
dalr_dvy = 1/vx_eff;
dalr_dr  = -lr/vx_eff;

dFyf = -Cf*[dalf_dvx; dalf_dvy; dalf_dr];
dFyr = -Cr*[dalr_dvx; dalr_dvy; dalr_dr];

% dvx
F(1,1) = 1 + Ts*(-sin(delta)*dFyf(1))/m;
F(1,2) = Ts*(r - sin(delta)*dFyf(2))/m;
F(1,3) = Ts*(vy - sin(delta)*dFyf(3))/m;
F(1,4) = Ts*(-alpha_f*sin(delta))/m;

% dvy
F(2,1) = Ts*(-r + cos(delta)*dFyf(1) + dFyr(1))/m;
F(2,2) = 1 + Ts*(cos(delta)*dFyf(2) + dFyr(2))/m;
F(2,3) = Ts*( -vx + cos(delta)*dFyf(3) + dFyr(3))/m;
F(2,4) = Ts*(-alpha_f*cos(delta))/m;
F(2,5) = Ts*(-alpha_r)/m;

% dr
F(3,1) = Ts*(lf*cos(delta)*dFyf(1) - lr*dFyr(1))/Jz;
F(3,2) = Ts*(lf*cos(delta)*dFyf(2) - lr*dFyr(2))/Jz;
F(3,3) = 1 + Ts*(lf*cos(delta)*dFyf(3) - lr*dFyr(3))/Jz;
F(3,4) = Ts*(-lf*alpha_f*cos(delta))/Jz;
F(3,5) = Ts*(lr*alpha_r)/Jz;

%% ---------------- Covariance prediction ----------------
P_pred = F*Pk*F' + Q;

%% ---------------- Measurement model ----------------
ax_hat = dvx - vy*r;                % longitudinal accel
ay_hat = dvy + vx*r;                % lateral accel
vx_hat = vx;
vy_hat = vy;
r_hat  = r;
wL_hat = (vx - track/2 * r)/Rw;
wR_hat = (vx + track/2 * r)/Rw;

z_hat = [ax_hat; ay_hat; vx_hat; vy_hat; r_hat; wL_hat; wR_hat];

%% ---------------- Measurement Jacobian H ----------------
H = zeros(7,5);

% ax = dvx - vy*r
H(1,1) = 0; % optional: include dvx derivative
H(1,2) = -r;
H(1,3) = -vy;

% ay = dvy + vx*r
H(2,1) = r;
H(2,2) = 1;
H(2,3) = vx;
H(2,4) = -alpha_f*cos(delta)/m;
H(2,5) = -alpha_r/m;

% vx
H(3,1) = 1;

% vy
H(4,2) = 1;

% r
H(5,3) = 1;

% wheel speeds
H(6,1) = 1/Rw;
H(6,3) = -track/(2*Rw);

H(7,1) = 1/Rw;
H(7,3) = track/(2*Rw);

%% ---------------- EKF update ----------------
S = H*P_pred*H' + R;
K = P_pred*H'/S;

x = x_pred + K*(z - z_hat);
Pk = (eye(5) - K*H)*P_pred;

%% ---------------- Output ----------------
xhat = x;
P = Pk;

end
